simulink model "PassVeh7DOF"  (R2019b)
settings: Solver=ode23tb  StartTime=0.0  StopTime=inf  FixedStep=.001  RelTol=3e-3
model workspace (MAT data in the model file):
  A_mu = 10
  B_reff = 8.386
  CONVERTER_DATA = [0 0.1 0.2 0.3 0.4 0.5 0.6 0.7 0.8 0.81 0.82 0.83 ... (63 elements, 21x3)]
  Cps = 2
  Cz = 7766.25
  DOWN_TABLE = [0 0 0 0 0 0 5 5 7.5 7.5 15 15 ... (30 elements, 6x5)]
  DOWN_TH_BP = [0 5 40 50 90 100]
  D_reff = 0.25826
  EMAP = [-40 215 245 264 264 267 267 267 267 267 -44 117 ... (110 elements, 10x11)]
  F0z = [6086.4 4324.8]
  F_reff = 0.07394
  F_zmax = 10000
  F_zmin = 100
  F_zo = 4000
  Kz = 48000
  MF : object (value not decoded)
  NCyl = 6
  NE_VEC = [800 1200 1600 2000 2400 2800 3200 3600 4000 4400 4800]
  Pstd = 101325
  Rair = 287
  SUS : object (value not decoded)
  TH_VEC = [0; 20; 30; 40; 50; 60; 70; 80; 90; 100]
  TWAITdn = 1.25
  TWAITup = 0.1
  Tin = [1 2 3 4 5 6 7 8 9 10 2 2 ... (20 elements, 10x2)]
  Tstd = 293.15
  UP_TABLE = [7.5 7.5 15 25 40 40 25 25 35 45 70 80 ... (30 elements, 6x5)]
  UP_TH_BP = [0 25 35 50 90 100]
  VEH : object (value not decoded)
  V_o = 16.7
  V_xlow = 1
  Vd = 0.00346
  WH : object (value not decoded)
  a = 1.515
  alpha_max = 1.5
  alpha_min = -1.5
  b = 1.504
  c_zo = 209651
  epsilon = 0.1
  f_air = [0 0 0 0 0 0 0 0 0 0 0 0 ... (256 elements, 16x16)]
  f_co = [0 0 0 0 0 0 0 0 0 0 0 0 ... (256 elements, 16x16)]
  f_co2 = [0 0 0 0 0 0 0 0 0 0 0 0 ... (256 elements, 16x16)]
  f_eff = [352.135682859 352.135682859 320.724378192 303.655312657 295.930136708 291.240087194 291.240271258 291.240312459 291.240275452 291.240198499 291.240100781 291.240018769 ... (256 elements, 16x16)]
  f_fuel = [0 0 0 0 0 0 0 0 0 0 0 0 ... (256 elements, 16x16)]
  f_hc = [0 0 0 0 0 0 0 0 0 0 0 0 ... (256 elements, 16x16)]
  f_nox = [0 0 0 0 0 0 0 0 0 0 0 0 ... (256 elements, 16x16)]
  f_pm = [0 0 0 0 0 0 0 0 0 0 0 0 ... (256 elements, 16x16)]
  f_susp_axl_bp = [1 2]
  f_susp_dz_bp = [-4 -0.14 -0.13 -0.12 -0.11 -0.1 -0.09 -0.08 -0.07 -0.06 -0.05 -0.04 ... (31 elements, 1x31)]
  f_susp_dzdot_bp = [-4 -0.14 -0.13 -0.12 -0.11 -0.1 -0.09 -0.08 -0.07 -0.06 -0.05 -0.04 ... (31 elements, 1x31)]
  f_susp_fmz = [-213379.591456 -28099.591456 -27619.591456 -27139.591456 -26659.591456 -26179.591456 -25699.591456 -25219.591456 -24739.591456 -24259.591456 -23779.591456 -23299.591456 ... (468968 elements, 31x31x61x2x4)]
  f_susp_geom = [-0.832564012244 0.043269987756 0.045538987756 0.047807987756 0.050076987756 0.052345987756 0.054614987756 0.056883987756 0.059152987756 0.061421987756 0.063690987756 0.065959987756 ... (11346 elements, 31x61x2x3)]
  f_susp_strgdelta_bp = [-0.523598775598 -0.506145483078 -0.488692190558 -0.471238898038 -0.453785605519 -0.436332312999 -0.418879020479 -0.401425727959 -0.383972435439 -0.366519142919 -0.349065850399 -0.331612557879 ... (61 elements, 1x61)]
  f_tbrake = [0 76.8593923996 105.140482948 131.533638111 157.926793274 176.658631717 176.65727296 176.656856686 176.656879077 176.657093756 176.657404516 176.65772406 ... (256 elements, 16x16)]
  f_tbrake_n_bpt = [0 649.519052838 912.419621844 1175.32019085 1438.22075986 1701.12132886 1964.02189787 2226.92246687 2489.82303588 2752.72360489 3015.62417389 3278.5247429 ... (16 elements, 1x16)]
  f_tbrake_t_bpt = [0 34.6410161514 61.0341713143 87.4273264773 113.82048164 140.213636803 166.606791966 192.999947129 219.393102292 245.786257455 272.179412618 298.572567781 ... (16 elements, 1x16)]
  f_texh = [766.752464599 766.752464599 786.17542386 801.679939032 884.591982581 910.574397722 910.571871054 910.570774534 910.570601632 910.570821151 910.571247242 910.571639815 ... (256 elements, 16x16)]
  f_twc_eff_co = [0.17 0.25 0.45 0.99 0.99 0.99 0.99]
  f_twc_eff_hc = [0.21 0.375 0.75 0.98 0.98 0.98 0.98]
  f_twc_eff_lam = [0.909090909 0.944055944 0.979020979 1 1.013986014 1.048951049 1.083916084]
  f_twc_eff_nox = [0.98 0.98 0.98 0.97 0.05 0.02 0]
  h = 0.134
  k_z = 50
  kappa_max = 1.5
  kappa_min = -1.5
  lam_Cx = 1
  lam_Cy = 1
  lam_Cz = 1
  lam_Ex = 1
  lam_Ey = 1
  lam_F_zo = 1
  lam_Hx = 1
  lam_Hy = 1
  lam_Kxkappa = 1
  lam_Kyalpha = 1
  lam_Kygamma = 1
  lam_Kzgamma = 1
  lam_Mr = 1
  lam_Mx = 1
  lam_My = 1
  lam_S = 1
  lam_VMx = 1
  lam_Vx = 1
  lam_Vy = 1
  lam_Vykappa = 1
  lam_muV = 0
  lam_mux = 1
  lam_muy = 1
  lam_t = 1
  lam_xalpha = 1
  lam_ykappa = 1
  numWheel = 4
  p_Cx1 = 1.579
  p_Cy1 = 1.3332
  p_Dx1 = 1.0422
  p_Dx2 = -0.08285
  p_Dx3 = 0
  p_Dy1 = 0.8784
  p_Dy2 = -0.06445
  p_Dy3 = 0
  p_Ex1 = 0.11185
  p_Ex2 = 0.3127
  p_Ex3 = 0
  p_Ex4 = 0.001603
  p_Ey1 = -0.8227
  p_Ey2 = -0.6062
  p_Ey3 = 0.09825
  p_Ey4 = -6.546
  p_Ey5 = 0
  p_Fz1 = 0.7098
  p_Hx1 = 0.00021585
  p_Hx2 = 0.0011538
  p_Hy1 = -0.0018043
  p_Hy2 = 0.003518
  p_Kx1 = 21.69
  p_Kx2 = 13.774
  p_Kx3 = -0.4119
  p_Ky1 = -15.314
  p_Ky2 = 1.7044
  p_Ky3 = 0.36986
  p_Ky4 = 1.9896
  p_Ky5 = 0
  p_Ky6 = -0.9004
  p_Ky7 = -0.2328
  p_Vx1 = 1.5973e-05
  p_Vx2 = 0.0001043
  p_Vy1 = -0.006642
  p_Vy2 = 0.03597
  p_Vy3 = -0.1621
  p_Vy4 = -0.4908
  p_pmx1 = 0
  p_px1 = -0.3489
  p_px2 = 0.382
  p_px3 = -0.09634
  p_px4 = 0.06447
  p_py1 = -0.6249
  p_py2 = -0.06535
  p_py3 = -0.1668
  p_py4 = 0.2834
  p_py5 = 0
  path : object (value not decoded)
  pio = 220000
  q_Fcx = 0
  q_Fz2 = 15.4
  q_Fzy = 0
  q_reo = 0.9974
  q_sx1 = -0.007764
  q_sx10 = 0.2824
  q_sx11 = 5.349
  q_sx12 = 0
  q_sx13 = 0
  q_sx14 = 0
  q_sx2 = 1.1915
  q_sx3 = 0.013948
  q_sx4 = 4.912
  q_sx5 = 1.02
  q_sx6 = 22.83
  q_sx7 = 0.7104
  q_sx8 = -0.023393
  q_sx9 = 0.6581
  q_sy1 = 0.00702
  q_sy2 = 0
  q_sy3 = 0.001515
  q_sy4 = 8.514e-05
  q_sy5 = 0
  q_sy6 = 0
  q_sy7 = 0.9008
  q_sy8 = -0.4089
  q_v1 = 0.0007742
  q_v2 = 0.04667
  r_Bx1 = 12.531
  r_Bx2 = 9.532
  r_Bx3 = 0
  r_By1 = 10.615
  r_By2 = 7.705
  r_By3 = 3.433e-06
  r_By4 = 0
  r_Cx1 = 1.019
  r_Cy1 = 1.0585
  r_Ex1 = -0.4487
  r_Ex2 = -0.4726
  r_Ey1 = 0.3132
  r_Ey2 = 7.63e-06
  r_Hx1 = 0.0002374
  r_Hy1 = 0.011646
  r_Hy2 = 7.63e-06
  r_Vy1 = 0.05654
  r_Vy2 = 7.63e-06
  r_Vy3 = 0
  r_Vy4 = 99.9
  r_Vy5 = 2
  r_Vy6 = 15.814
  r_o = 0.3135
  reqTmaxT = [nan 0.285774810084 0.647179872268 nan nan nan nan nan nan nan nan nan ... (168 elements, 21x8)]
  vehSpd = [0 2.77777777778 5.55555555556 8.33333333333 11.1111111111 13.8888888889 16.6666666667 19.4444444444 22.2222222222 25 27.7777777778 30.5555555556 ... (21 elements, 1x21)]
  vehWidth = 2
  w = 1
symbols that are objects in the model workspace (value not decoded): VEH
libraries: autolibshared x3, vehdynlibtirecommon x2, autolibutils x2, sharedtransform x1
(part 2 of 4)

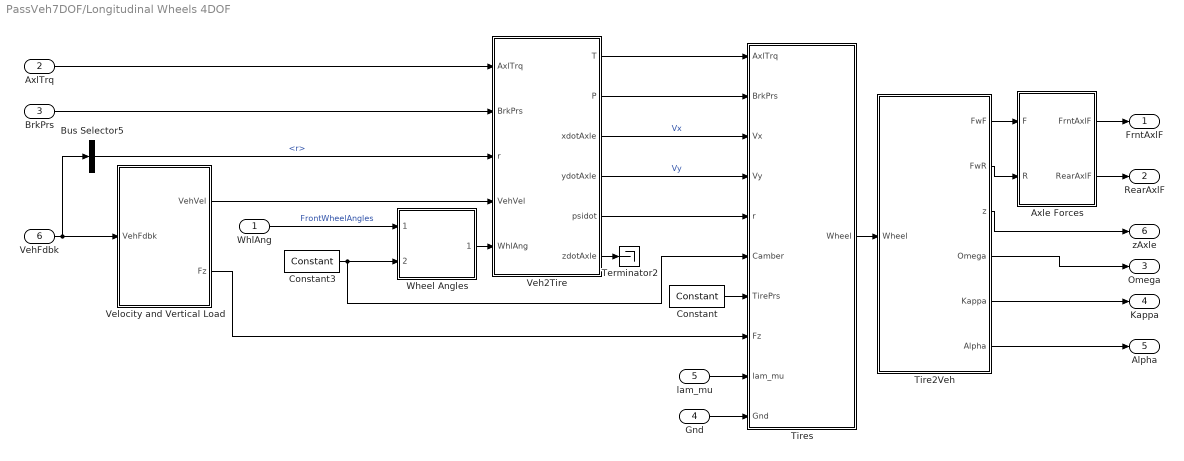
== system PassVeh7DOF/Longitudinal Wheels 4DOF ==
  WhlAng : Inport
  AxlTrq : Inport  Port=2
  BrkPrs : Inport  Port=3
  Gnd : Inport  Port=4  PortDimensions=4
  lam_mu : Inport  Port=5  PortDimensions=4
  VehFdbk : Inport  Port=6
  Axle Forces : Subsystem  VariantControlMode=Label  Variant=on  LabelModeActiveChoice=0
  Bus Selector5 : BusSelector  OutputSignals=BdyFrm.Cg.AngVel.r
  Constant : vehdynlibtirecommon/Constant  const=220000  numWheels=4
      settings: SourceProductName=Vehicle Dynamics Blockset  SourceProductBaseCode=VE
  Constant3 : vehdynlibtirecommon/Constant  const=0  numWheels=4
      settings: SourceProductName=Vehicle Dynamics Blockset  SourceProductBaseCode=VE
  Terminator2 : Terminator
  Tire2Veh : Subsystem
  Tires : Subsystem
  Veh2Tire : Subsystem
  Velocity and Vertical Load : Subsystem  VariantControlMode=Label  Variant=on  LabelModeActiveChoice=0
  Wheel Angles : Subsystem
  FrntAxlF : Outport  Unit=N  VectorParamsAs1DForOutWhenUnconnected=off
  RearAxlF : Outport  Port=2  Unit=N  VectorParamsAs1DForOutWhenUnconnected=off
  Omega : Outport  Port=3  VectorParamsAs1DForOutWhenUnconnected=off
  Kappa : Outport  Port=4  VectorParamsAs1DForOutWhenUnconnected=off
  Alpha : Outport  Port=5  VectorParamsAs1DForOutWhenUnconnected=off
  zAxle : Outport  Port=6  VectorParamsAs1DForOutWhenUnconnected=off
  wires:
  Wheel Angles/1(WhlAngB) -> Veh2Tire/5(WhlAng)
  Tires/1(Wheel) -> Tire2Veh/1(Wheel)
  lam_mu/1 -> Tires/9(lam_mu)
  Constant/1 -> Tires/7(TirePrs)
  Constant3/1 -> Wheel Angles/2(Camber), Tires/6(Camber)
  Veh2Tire/3(xdotAxle) -> Tires/3(Vx)  "Vx"
  Gnd/1 -> Tires/10(Gnd)
  VehFdbk/1 -> Bus Selector5/1, Velocity and Vertical Load/1(VehFdbk)
  AxlTrq/1 -> Veh2Tire/1(AxlTrq)
  Veh2Tire/1(T) -> Tires/1(AxlTrq)
  Veh2Tire/2(P) -> Tires/2(BrkPrs)
  BrkPrs/1 -> Veh2Tire/2(BrkPrs)
  Bus Selector5/1 -> Veh2Tire/3(r)  "<r>"
  Veh2Tire/6(zdotAxle) -> Terminator2/1
  WhlAng/1 -> Wheel Angles/1(WheelAng)  "FrontWheelAngles"
  Veh2Tire/4(ydotAxle) -> Tires/4(Vy)  "Vy"
  Veh2Tire/5(psidot) -> Tires/5(r)
  Velocity and Vertical Load/2(Fz) -> Tires/8(Fz)
  Velocity and Vertical Load/1(VehVel) -> Veh2Tire/4(VehVel)
  Axle Forces/1(FrntAxlF) -> FrntAxlF/1
  Axle Forces/2(RearAxlF) -> RearAxlF/1
  Tire2Veh/1(FwF) -> Axle Forces/1(F)
  Tire2Veh/2(FwR) -> Axle Forces/2(R)
  Tire2Veh/3(z) -> zAxle/1
  Tire2Veh/4(Omega) -> Omega/1
  Tire2Veh/5(Kappa) -> Kappa/1
  Tire2Veh/6(Alpha) -> Alpha/1

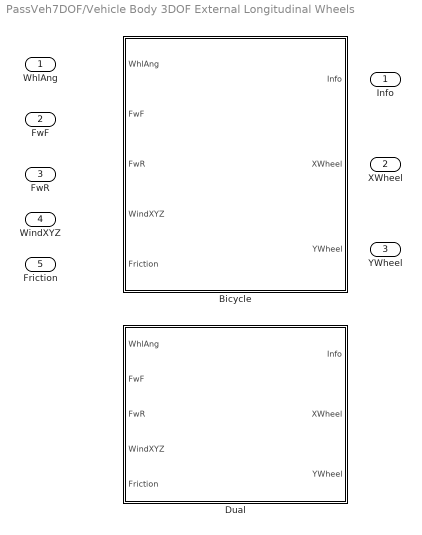
== system PassVeh7DOF/Vehicle Body 3DOF External Longitudinal Wheels ==
  WhlAng : Inport
  "FwF " : Inport  Port=2
  "FwR " : Inport  Port=3
  WindXYZ : Inport  Port=4
  Friction : Inport  Port=5  Unit=1  PortDimensions=4
  Bicycle : Subsystem  VariantControl=0
  Dual : Subsystem  VariantControl=1
  " Info" : Outport  VectorParamsAs1DForOutWhenUnconnected=off
  " XWheel" : Outport  Port=2  VectorParamsAs1DForOutWhenUnconnected=off
  " YWheel" : Outport  Port=3  VectorParamsAs1DForOutWhenUnconnected=off

== system PassVeh7DOF/Longitudinal Wheels 4DOF/Axle Forces ==
  note: 1) Add Subsystem or Model blocks as valid variant choices.
      | 2) You cannot connect blocks at this level. At simulation, connectivity is automatically
      | determined, based on the active variant and port name matching.
  F : Inport
  R : Inport  Port=2
  Bicycle : Subsystem  VariantControl=0
  Dual : Subsystem  VariantControl=1
  FrntAxlF : Outport  Unit=N  VectorParamsAs1DForOutWhenUnconnected=off
  RearAxlF : Outport  Port=2  Unit=N  VectorParamsAs1DForOutWhenUnconnected=off

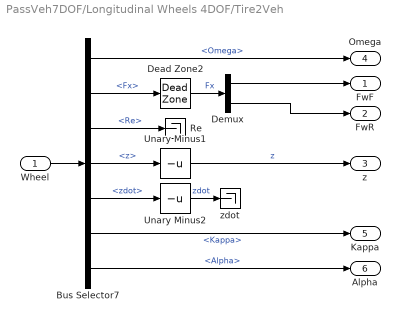
== system PassVeh7DOF/Longitudinal Wheels 4DOF/Tire2Veh ==
  Wheel : Inport
  Bus Selector7 : BusSelector  OutputSignals=Omega,Fx,Re,z,zdot,Kappa,Alpha
  Dead Zone2 : DeadZone  LowerValue=-5  UpperValue=5  ZeroCross=off  SaturateOnIntegerOverflow=on
  Demux : Demux  Outputs=[2,2]
  Re : Terminator
  Unary Minus1 : UnaryMinus
  Unary Minus2 : UnaryMinus
  zdot : Terminator
  FwF : Outport  VectorParamsAs1DForOutWhenUnconnected=off
  FwR : Outport  Port=2  VectorParamsAs1DForOutWhenUnconnected=off
  z : Outport  Port=3  VectorParamsAs1DForOutWhenUnconnected=off
  Omega : Outport  Port=4  VectorParamsAs1DForOutWhenUnconnected=off
  Kappa : Outport  Port=5  VectorParamsAs1DForOutWhenUnconnected=off
  Alpha : Outport  Port=6  VectorParamsAs1DForOutWhenUnconnected=off
  wires:
  Bus Selector7/2 -> Dead Zone2/1  "<Fx>"
  Dead Zone2/1 -> Demux/1  "Fx"
  Demux/1 -> FwF/1
  Wheel/1 -> Bus Selector7/1
  Bus Selector7/1 -> Omega/1  "<Omega>"
  Bus Selector7/5 -> Unary Minus2/1  "<zdot>"
  Bus Selector7/4 -> Unary Minus1/1  "<z>"
  Unary Minus1/1 -> z/1  "z"
  Demux/2 -> FwR/1
  Bus Selector7/6 -> Kappa/1  "<Kappa>"
  Unary Minus2/1 -> zdot/1  "zdot"
  Bus Selector7/3 -> Re/1  "<Re>"
  Bus Selector7/7 -> Alpha/1  "<Alpha>"

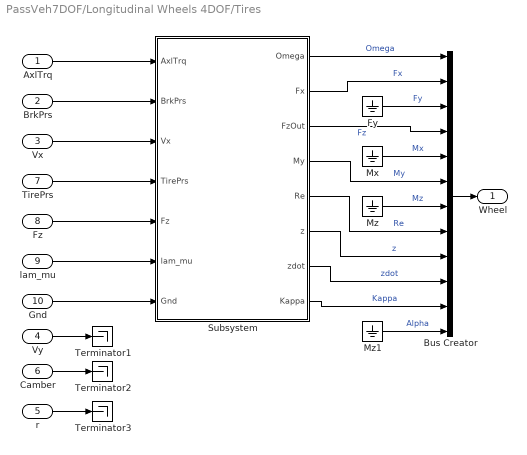
== system PassVeh7DOF/Longitudinal Wheels 4DOF/Tires ==
  AxlTrq : Inport
  BrkPrs : Inport  Port=2
  Vx : Inport  Port=3
  Vy : Inport  Port=4
  r : Inport  Port=5
  Camber : Inport  Port=6
  TirePrs : Inport  Port=7
  Fz : Inport  Port=8
  lam_mu : Inport  Port=9
  Gnd : Inport  Port=10
  Bus Creator : BusCreator  Inputs=12
  Fy : Ground
  Mx : Ground
  Mz : Ground
  Mz1 : Ground
  Subsystem : Subsystem
  Terminator1 : Terminator
  Terminator2 : Terminator
  Terminator3 : Terminator
  Wheel : Outport  VectorParamsAs1DForOutWhenUnconnected=off
  wires:
  Vy/1 -> Terminator1/1
  Camber/1 -> Terminator2/1
  r/1 -> Terminator3/1
  Bus Creator/1 -> Wheel/1
  Subsystem/7(zdot) -> Bus Creator/10  "zdot"
  Subsystem/6(z) -> Bus Creator/9  "z"
  Subsystem/2(Fx) -> Bus Creator/2  "Fx"
  Subsystem/1(Omega) -> Bus Creator/1  "Omega"
  Subsystem/5(Re) -> Bus Creator/8  "Re"
  Subsystem/3(FzOut) -> Bus Creator/4  "Fz"
  Subsystem/4(My) -> Bus Creator/6  "My"
  Fy/1 -> Bus Creator/3  "Fy"
  Mx/1 -> Bus Creator/5  "Mx"
  Mz/1 -> Bus Creator/7  "Mz"
  Subsystem/8(Kappa) -> Bus Creator/11  "Kappa"
  Mz1/1 -> Bus Creator/12  "Alpha"
  AxlTrq/1 -> Subsystem/1(AxlTrq)
  BrkPrs/1 -> Subsystem/2(BrkPrs)
  Vx/1 -> Subsystem/3(Vx)
  TirePrs/1 -> Subsystem/4(TirePrs)
  Fz/1 -> Subsystem/5(Fz)
  lam_mu/1 -> Subsystem/6(lam_mu)
  Gnd/1 -> Subsystem/7(Gnd)

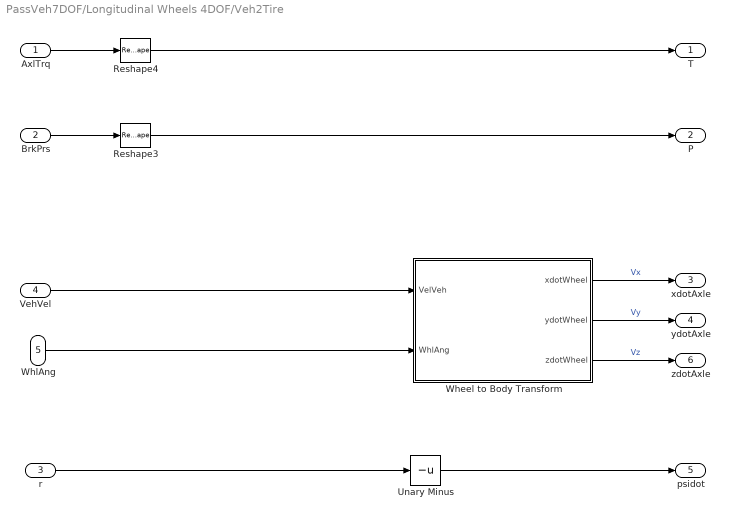
== system PassVeh7DOF/Longitudinal Wheels 4DOF/Veh2Tire ==
  AxlTrq : Inport
  BrkPrs : Inport  Port=2
  r : Inport  Port=3
  VehVel : Inport  Port=4
  WhlAng : Inport  Port=5
  Reshape3 : Reshape
  Reshape4 : Reshape
  Unary Minus : UnaryMinus
  Wheel to Body Transform : Subsystem
  T : Outport  VectorParamsAs1DForOutWhenUnconnected=off
  P : Outport  Port=2  VectorParamsAs1DForOutWhenUnconnected=off
  xdotAxle : Outport  Port=3  VectorParamsAs1DForOutWhenUnconnected=off
  ydotAxle : Outport  Port=4  VectorParamsAs1DForOutWhenUnconnected=off
  psidot : Outport  Port=5  VectorParamsAs1DForOutWhenUnconnected=off
  zdotAxle : Outport  Port=6  VectorParamsAs1DForOutWhenUnconnected=off
  wires:
  BrkPrs/1 -> Reshape3/1
  AxlTrq/1 -> Reshape4/1
  Wheel to Body Transform/1(xdotWheel) -> xdotAxle/1  "Vx"
  Wheel to Body Transform/2(ydotWheel) -> ydotAxle/1  "Vy"
  r/1 -> Unary Minus/1
  Reshape4/1 -> T/1
  VehVel/1 -> Wheel to Body Transform/1(VelVeh)
  WhlAng/1 -> Wheel to Body Transform/2(WhlAng)
  Wheel to Body Transform/3(zdotWheel) -> zdotAxle/1  "Vz"
  Unary Minus/1 -> psidot/1
  Reshape3/1 -> P/1

== system PassVeh7DOF/Longitudinal Wheels 4DOF/Velocity and Vertical Load ==
  note: 1) Add Subsystem or Model blocks as valid variant choices.
      | 2) You cannot connect blocks at this level. At simulation, connectivity is automatically
      | determined, based on the active variant and port name matching.
  VehFdbk : Inport
  Bicycle : Subsystem  VariantControl=0
  Dual : Subsystem  VariantControl=1
  VehVel : Outport  VectorParamsAs1DForOutWhenUnconnected=off
  Fz : Outport  Port=2  PortDimensions=4  VectorParamsAs1DForOutWhenUnconnected=off

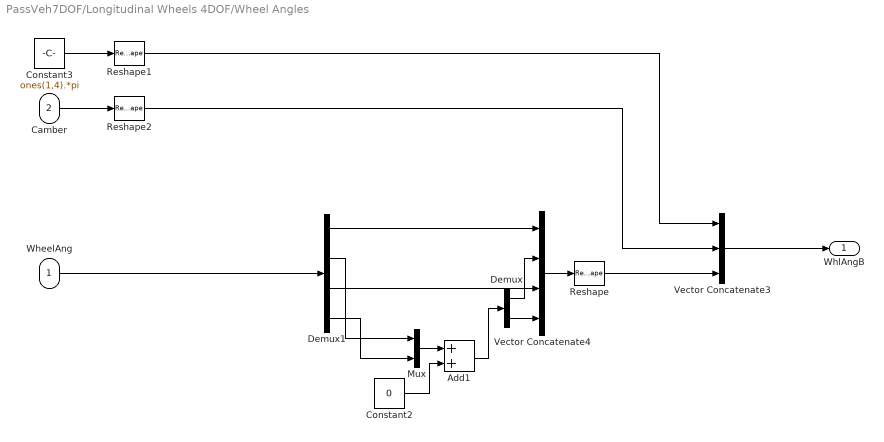
== system PassVeh7DOF/Longitudinal Wheels 4DOF/Wheel Angles ==
  WheelAng : Inport
  Camber : Inport  Port=2
  Add1 : Sum
  Constant2 : Constant  Value=0
  Constant3 : Constant  Value=ones(1,4).*pi
  Demux : Demux  Outputs=2
  Demux1 : Demux
  Mux : Mux  Inputs=2
  Reshape : Reshape  OutputDimensionality=Row vector (2-D)
  Reshape1 : Reshape  OutputDimensionality=Row vector (2-D)
  Reshape2 : Reshape  OutputDimensionality=Row vector (2-D)
  Vector Concatenate3 : Concatenate  NumInputs=3  Mode=Multidimensional array
  Vector Concatenate4 : Concatenate  NumInputs=4
  WhlAngB : Outport  VectorParamsAs1DForOutWhenUnconnected=off
  wires:
  Demux1/2 -> Mux/1
  Constant2/1 -> Add1/2
  Add1/1 -> Demux/1
  Demux1/3 -> Vector Concatenate4/3
  Demux1/1 -> Vector Concatenate4/1
  Mux/1 -> Add1/1
  Demux1/4 -> Mux/2
  Demux/1 -> Vector Concatenate4/2
  Demux/2 -> Vector Concatenate4/4
  Vector Concatenate4/1 -> Reshape/1
  Constant3/1 -> Reshape1/1
  Vector Concatenate3/1 -> WhlAngB/1
  Reshape/1 -> Vector Concatenate3/3
  Reshape1/1 -> Vector Concatenate3/1
  Reshape2/1 -> Vector Concatenate3/2
  Camber/1 -> Reshape2/1
  WheelAng/1 -> Demux1/1

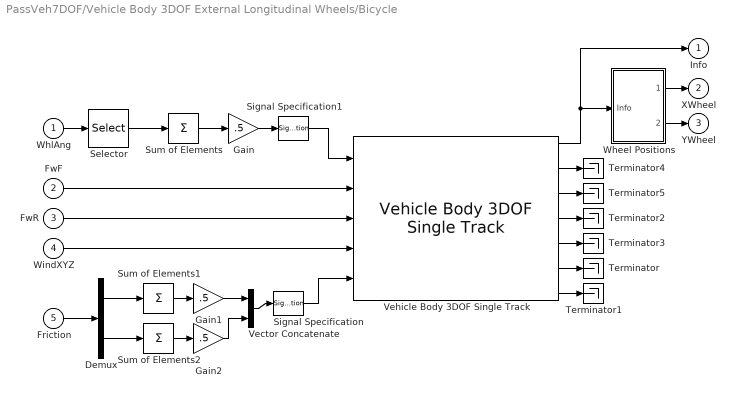
== system PassVeh7DOF/Vehicle Body 3DOF External Longitudinal Wheels/Bicycle ==
  WhlAng : Inport
  "FwF " : Inport  Port=2
  "FwR " : Inport  Port=3
  WindXYZ : Inport  Port=4
  Friction : Inport  Port=5
  Demux : Demux  Outputs=[2,2]
  Gain : Gain  Gain=.5
  Gain1 : Gain  Gain=.5
  Gain2 : Gain  Gain=.5
  Selector : Selector  InputPortWidth=4  IndexOptions=Index vector (dialog)  Indices=[1 2]  OutputSizes=1
  Signal Specification : SignalSpecification  Unit=1
  Signal Specification1 : SignalSpecification  Unit=rad
  Sum of Elements : Sum  Inputs=+
  Sum of Elements1 : Sum  Inputs=+
  Sum of Elements2 : Sum  Inputs=+
  Terminator{,1..5} (6 alike) : Terminator
  Vector Concatenate : Concatenate
  Vehicle Body 3DOF Single Track : autolibshared/Vehicle Body 3DOF Single Track  trackMode=Single (bicycle)  inputMode=External longitudinal forces  frontSteerMode=on  rearSteerMode=off  windMode=on  muMode=on  extFMode=off  extMMode=off  extXo=off  extpsio=off  extxdoto=off  extro=off  extYo=off  extTamb=off  extydoto=off  aMode=2  NF=VEH.NumberOfWheelsPerAxle  NR=VEH.NumberOfWheelsPerAxle  m=VEH.Mass  a=VEH.FrontAxlePositionfromCG  b=VEH.RearAxlePositionfromCG  h=VEH.HeightCG  X_o=VEH.InitialLongPosition  xdot_o=VEH.InitialLongVel  CalphaMode=off  sigmaMode=on  d=0  w=1.922.*[1 1]  Cy_f=15000  Cy_r=35000  sigma_f=.1  sigma_r=.1  alpha_f_brk=[-.1 .1]  Cy_f_data=[-9e3 9e3]  alpha_r_brk=[-.1 .1]  Cy_r_data=[-9e3 9e3]  Y_o=VEH.InitialLatPosition  ydot_o=VEH.InitialLatVel  Izz=VEH.YawMomentInertia  psi_o=VEH.InitialYawAngle  r_o=VEH.InitialYawRate  Af=VEH.FrontalArea  Cd=.3  Cl=.1  Cpm=.1  beta_w=[0:0.01:0.3]  Cs=[0:0.03:0.9]  Cym=[0:0.01:0.3]  Pabs=101325  Tair=273  g=9.81  mu=1  xdot_tol=1  Fznom=5000  Fxtire_sat=7e3*1e3  Fytire_sat=2e3*1e3  longOff=0  latOff=0  vertOff=.0112  wrapAng=off
      settings: SourceProductName=Powertrain Blockset  SourceProductBaseCode=PW
  Wheel Positions : Subsystem
  " Info" : Outport  VectorParamsAs1DForOutWhenUnconnected=off
  XWheel : Outport  Port=2  Unit=m  VectorParamsAs1DForOutWhenUnconnected=off
  " YWheel" : Outport  Port=3  Unit=m  VectorParamsAs1DForOutWhenUnconnected=off
  wires:
  "FwR "/1 -> Vehicle Body 3DOF Single Track/3
  "FwF "/1 -> Vehicle Body 3DOF Single Track/2
  Vehicle Body 3DOF Single Track/1 -> " Info"/1, Wheel Positions/1(Info)
  WhlAng/1 -> Selector/1
  Gain/1 -> Signal Specification1/1
  Sum of Elements/1 -> Gain/1
  Vehicle Body 3DOF Single Track/6 -> Terminator/1
  Vehicle Body 3DOF Single Track/7 -> Terminator1/1
  WindXYZ/1 -> Vehicle Body 3DOF Single Track/4
  Selector/1 -> Sum of Elements/1
  Demux/1 -> Sum of Elements1/1
  Friction/1 -> Demux/1
  Sum of Elements1/1 -> Gain1/1
  Sum of Elements2/1 -> Gain2/1
  Demux/2 -> Sum of Elements2/1
  Gain1/1 -> Vector Concatenate/1
  Gain2/1 -> Vector Concatenate/2
  Vector Concatenate/1 -> Signal Specification/1
  Signal Specification/1 -> Vehicle Body 3DOF Single Track/5
  Signal Specification1/1 -> Vehicle Body 3DOF Single Track/1
  Wheel Positions/2(YWheel) -> " YWheel"/1
  Wheel Positions/1(XWheel) -> XWheel/1
  Vehicle Body 3DOF Single Track/4 -> Terminator2/1
  Vehicle Body 3DOF Single Track/5 -> Terminator3/1
  Vehicle Body 3DOF Single Track/2 -> Terminator4/1
  Vehicle Body 3DOF Single Track/3 -> Terminator5/1

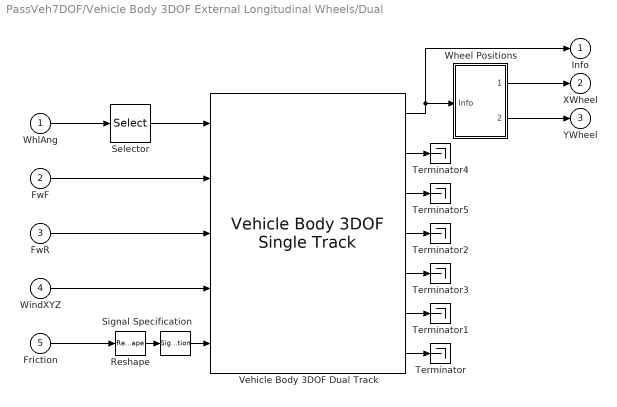
== system PassVeh7DOF/Vehicle Body 3DOF External Longitudinal Wheels/Dual ==
  WhlAng : Inport
  "FwF " : Inport  Port=2
  "FwR " : Inport  Port=3
  WindXYZ : Inport  Port=4
  Friction : Inport  Port=5
  Reshape : Reshape  OutputDimensionality=Customize  OutputDimensions=[2,2]
  Selector : Selector  InputPortWidth=4  IndexOptions=Index vector (dialog)  Indices=[1 2]  OutputSizes=1
  Signal Specification : SignalSpecification  Unit=1
  Terminator{,1..5} (6 alike) : Terminator
  Vehicle Body 3DOF Dual Track : autolibshared/Vehicle Body 3DOF Single Track  trackMode=Dual  inputMode=External longitudinal forces  frontSteerMode=on  rearSteerMode=off  windMode=on  muMode=on  extFMode=off  extMMode=off  extXo=off  extpsio=off  extxdoto=off  extro=off  extYo=off  extTamb=off  extydoto=off  aMode=2  NF=VEH.NumberOfWheelsPerAxle  NR=VEH.NumberOfWheelsPerAxle  m=VEH.Mass  a=VEH.FrontAxlePositionfromCG  b=VEH.RearAxlePositionfromCG  h=VEH.HeightCG  X_o=VEH.InitialLongPosition  xdot_o=VEH.InitialLatVel  CalphaMode=off  sigmaMode=on  d=0  w=VEH.TrackWidth.*[1 1]  Cy_f=15000  Cy_r=35000  sigma_f=.1  sigma_r=.1  alpha_f_brk=[-.1 .1]  Cy_f_data=[-9e3 9e3]  alpha_r_brk=[-.1 .1]  Cy_r_data=[-9e3 9e3]  Y_o=VEH.InitialLatPosition  ydot_o=VEH.InitialLatVel  Izz=VEH.YawMomentInertia  psi_o=VEH.InitialYawAngle  r_o=VEH.InitialYawRate  Af=VEH.FrontalArea  Cd=.3  Cl=.1  Cpm=.1  beta_w=[0:0.01:0.3]  Cs=[0:0.03:0.9]  Cym=[0:0.01:0.3]  Pabs=101325  Tair=273  g=9.81  mu=1  xdot_tol=1  Fznom=5000  Fxtire_sat=7e3*1e3  Fytire_sat=2e3*1e3  longOff=0  latOff=0  vertOff=.0112  wrapAng=off
      settings: SourceProductName=Powertrain Blockset  SourceProductBaseCode=PW
  Wheel Positions : Subsystem
  " Info" : Outport  VectorParamsAs1DForOutWhenUnconnected=off
  " XWheel" : Outport  Port=2  VectorParamsAs1DForOutWhenUnconnected=off
  " YWheel" : Outport  Port=3  VectorParamsAs1DForOutWhenUnconnected=off
  wires:
  WhlAng/1 -> Selector/1
  Selector/1 -> Vehicle Body 3DOF Dual Track/1
  Friction/1 -> Reshape/1
  Reshape/1 -> Signal Specification/1
  Vehicle Body 3DOF Dual Track/1 -> " Info"/1, Wheel Positions/1(Info)
  Wheel Positions/1(XWheel) -> " XWheel"/1
  Wheel Positions/2(YWheel) -> " YWheel"/1
  Vehicle Body 3DOF Dual Track/2 -> Terminator4/1
  Vehicle Body 3DOF Dual Track/3 -> Terminator5/1
  Vehicle Body 3DOF Dual Track/6 -> Terminator1/1
  Vehicle Body 3DOF Dual Track/4 -> Terminator2/1
  Vehicle Body 3DOF Dual Track/5 -> Terminator3/1
  Vehicle Body 3DOF Dual Track/7 -> Terminator/1
  Signal Specification/1 -> Vehicle Body 3DOF Dual Track/5
  WindXYZ/1 -> Vehicle Body 3DOF Dual Track/4
  "FwF "/1 -> Vehicle Body 3DOF Dual Track/2
  "FwR "/1 -> Vehicle Body 3DOF Dual Track/3

== system PassVeh7DOF/Longitudinal Wheels 4DOF/Axle Forces/Bicycle ==
  F : Inport
  R : Inport  Port=2
  Sum of Elements : Sum  Inputs=+
  Sum of Elements1 : Sum  Inputs=+
  FrntAxlF : Outport  Unit=N  VectorParamsAs1DForOutWhenUnconnected=off
  RearAxlF : Outport  Port=2  Unit=N  VectorParamsAs1DForOutWhenUnconnected=off
  wires:
  Sum of Elements/1 -> FrntAxlF/1
  Sum of Elements1/1 -> RearAxlF/1
  R/1 -> Sum of Elements1/1
  F/1 -> Sum of Elements/1

== system PassVeh7DOF/Longitudinal Wheels 4DOF/Axle Forces/Dual ==
  F : Inport
  R : Inport  Port=2
  FrntAxlF : Outport  Unit=N  VectorParamsAs1DForOutWhenUnconnected=off
  RearAxlF : Outport  Port=2  Unit=N  VectorParamsAs1DForOutWhenUnconnected=off
  wires:
  R/1 -> RearAxlF/1
  F/1 -> FrntAxlF/1
